simulink model "Motor3_Avellaneda"  (R2023b)
settings: Solver=VariableStepAuto  StartTime=0.0  StopTime=3  FixedStep=1  MaxStep=0.00001  RelTol=1e-3
libraries: simulink x2
settings Model: Creator=Usuario  LastModifiedBy=Usuario

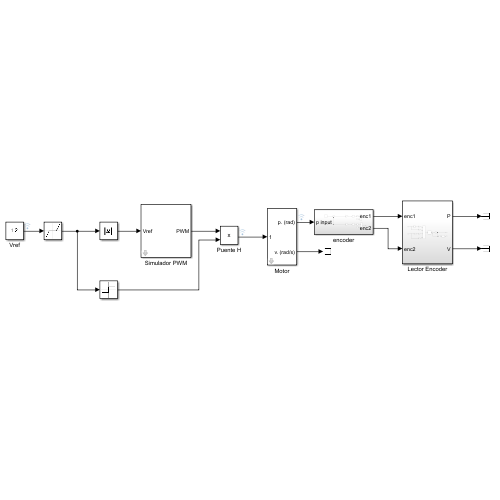
[thumbnail: Simulink's stored preview of the top-level diagram]
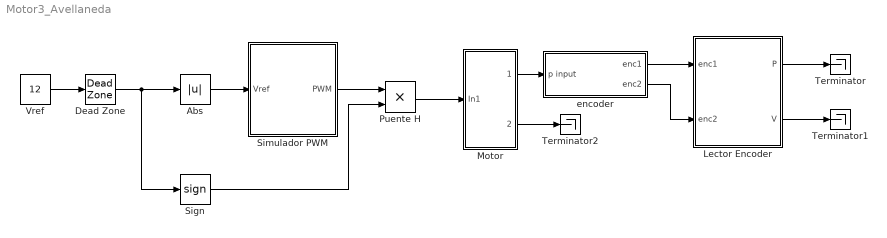
== system Motor3_Avellaneda ==
  Abs : Abs  SaturateOnIntegerOverflow=off
  Dead Zone : DeadZone  LowerValue=0  UpperValue=0
  Lector Encoder : Subsystem
  Motor : Subsystem  mask{Parameter1=61.441545, Parameter2=6215.39669}
      mask prompts: Parameter1 "p"; Parameter2 "K_e"
  Puente H : Product
  Sign : Signum
  Simulador PWM : Subsystem  mask{T=0.001, Vmax=12}
      mask prompts: T "Periodo T"; Vmax "Voltaje de la fuente Vmax"
  Terminator : Terminator
  Terminator1 : Terminator
  Terminator2 : Terminator
  Vref : Constant  Value=12
  encoder : Subsystem
  wires:
  Abs/1 -> Simulador PWM/1(Vref)
  Sign/1 -> Puente H/2
  Dead Zone/1 -> Sign/1, Abs/1
  Lector Encoder/2(V) -> Terminator1/1
  Simulador PWM/1(PWM) -> Puente H/1
  Motor/2(v. (rad/s)) -> Terminator2/1
  Motor/1(p. (rad)) -> encoder/1(p input)
  encoder/1(enc1) -> Lector Encoder/1(enc1)
  encoder/2(enc2) -> Lector Encoder/2(enc2)
  Lector Encoder/1(P) -> Terminator/1
  Vref/1 -> Dead Zone/1
  Puente H/1 -> Motor/1(In1)

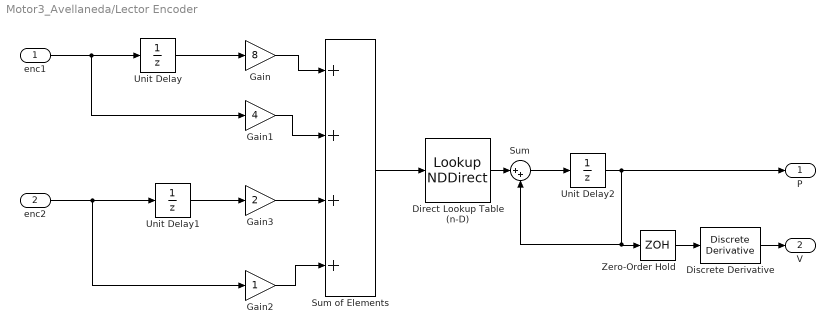
== system Motor3_Avellaneda/Lector Encoder ==
  enc1 : Inport
  enc2 : Inport  Port=2
  Direct Lookup Table (n-D) : LookupNDDirect  NumberOfTableDimensions=1  Table=[0,-1,1,0,1,0,0,-1,-1,0,0,1,0,1,-1,0]
  Discrete Derivative : simulink/Discrete/Discrete Derivative  gainval=1.0  ICPrevScaledInput=0.0  OutMin=[]  OutMax=[]  OutDataType=fixdt(1, 16)  OutScaling=2^-10  DoSatur=off
  Gain : Gain  Gain=8
  Gain1 : Gain  Gain=4
  Gain2 : Gain
  Gain3 : Gain  Gain=2
  Sum : Sum  Inputs=|++
  Sum of Elements : Sum  Inputs=++++  OutDataTypeStr=double
  Unit Delay : UnitDelay  SampleTime=-1  HasFrameUpgradeWarning=on
  Unit Delay1 : UnitDelay  SampleTime=-1  HasFrameUpgradeWarning=on
  Unit Delay2 : UnitDelay  SampleTime=-1  HasFrameUpgradeWarning=on
  Zero-Order Hold : ZeroOrderHold  SampleTime=0.01
  P : Outport
  V : Outport  Port=2
  wires:
  enc1/1 -> Gain1/1, Unit Delay/1
  enc2/1 -> Gain2/1, Unit Delay1/1
  Unit Delay/1 -> Gain/1
  Unit Delay1/1 -> Gain3/1
  Gain/1 -> Sum of Elements/1
  Gain1/1 -> Sum of Elements/2
  Gain3/1 -> Sum of Elements/3
  Gain2/1 -> Sum of Elements/4
  Sum of Elements/1 -> Direct Lookup Table (n-D)/1
  Direct Lookup Table (n-D)/1 -> Sum/1
  Sum/1 -> Unit Delay2/1
  Unit Delay2/1 -> Sum/2, Zero-Order Hold/1, P/1
  Discrete Derivative/1 -> V/1
  Zero-Order Hold/1 -> Discrete Derivative/1

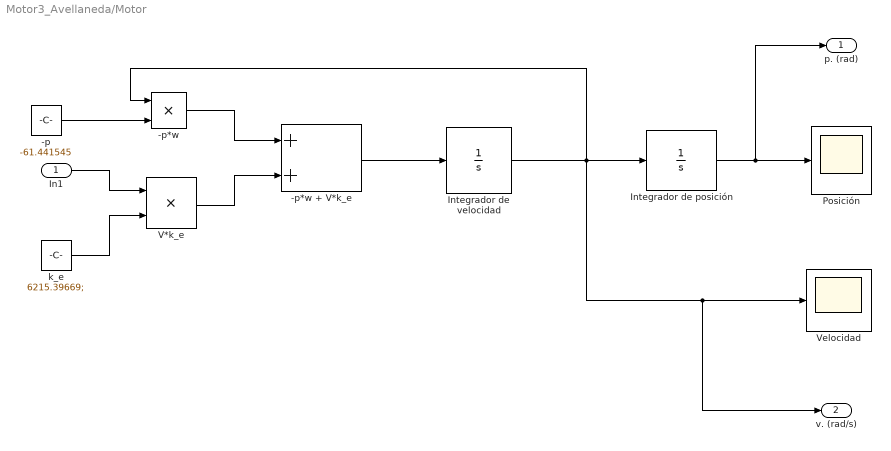
== system Motor3_Avellaneda/Motor ==
  In1 : Inport
  -p : Constant  Value=-61.441545
  -p*w : Product
  -p*w + V*k_e : Sum
  Integrador de posición : Integrator
  Integrador de velocidad : Integrator
  Posición : Scope
  V*k_e : Product
  Velocidad : Scope
  k_e : Constant  Value=6215.39669;
  p. (rad) : Outport
  v. (rad/s) : Outport  Port=2
  wires:
  Integrador de velocidad/1 -> -p*w/1, Integrador de posición/1, v. (rad/s)/1, Velocidad/1
  -p/1 -> -p*w/2
  Integrador de posición/1 -> Posición/1, p. (rad)/1
  -p*w + V*k_e/1 -> Integrador de velocidad/1
  -p*w/1 -> -p*w + V*k_e/1
  V*k_e/1 -> -p*w + V*k_e/2
  k_e/1 -> V*k_e/2
  In1/1 -> V*k_e/1

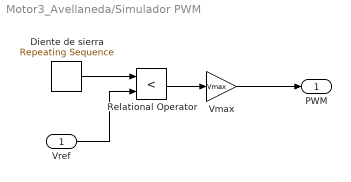
== system Motor3_Avellaneda/Simulador PWM ==
  Vref : Inport
  Diente de sierra : simulink/Sources/Repeating Sequence  rep_seq_t=linspace(0,T,100)  rep_seq_y=linspace(0,Vmax,100)
  Relational Operator : RelationalOperator  Operator=<  OutDataTypeStr=boolean  RndMeth=Simplest  InputSameDT=off
  Vmax : Gain  Gain=Vmax
  PWM : Outport
  wires:
  Vref/1 -> Relational Operator/2
  Relational Operator/1 -> Vmax/1
  Vmax/1 -> PWM/1
  Diente de sierra/1 -> Relational Operator/1

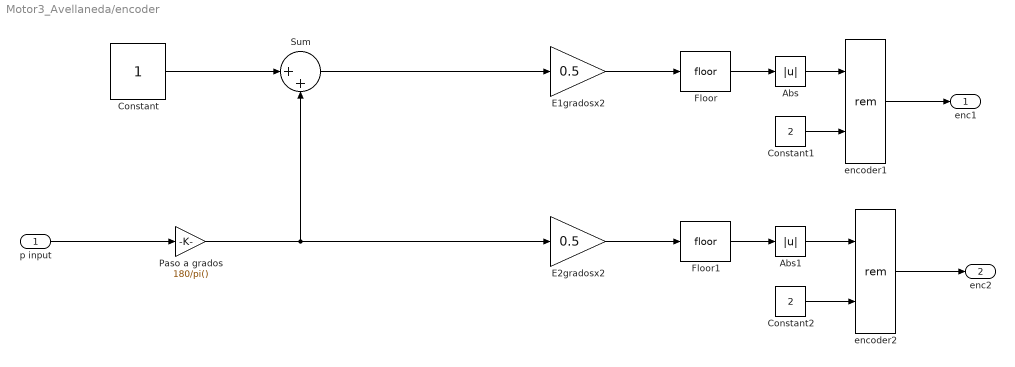
== system Motor3_Avellaneda/encoder ==
  p input : Inport
  Abs : Abs  SaturateOnIntegerOverflow=off
  Abs1 : Abs  SaturateOnIntegerOverflow=off
  Constant : Constant
  Constant1 : Constant  Value=2
  Constant2 : Constant  Value=2
  E1gradosx2 : Gain  Gain=0.5
  E2gradosx2 : Gain  Gain=0.5
  Floor : Rounding
  Floor1 : Rounding
  Paso a grados : Gain  Gain=180/pi()
  Sum : Sum  Inputs=|++
  encoder1 : Math  Operator=rem
  encoder2 : Math  Operator=rem
  enc1 : Outport
  enc2 : Outport  Port=2
  wires:
  Constant/1 -> Sum/1
  p input/1 -> Paso a grados/1
  Sum/1 -> E1gradosx2/1
  Paso a grados/1 -> Sum/2, E2gradosx2/1
  E1gradosx2/1 -> Floor/1
  E2gradosx2/1 -> Floor1/1
  Floor/1 -> Abs/1
  Floor1/1 -> Abs1/1
  Abs/1 -> encoder1/1
  Constant1/1 -> encoder1/2
  Abs1/1 -> encoder2/1
  Constant2/1 -> encoder2/2
  encoder1/1 -> enc1/1
  encoder2/1 -> enc2/1
